simulink model "commhdlPRBSLoopback"  (R2025b)
settings: Solver=FixedStepDiscrete  StartTime=0.0  StopTime=5000  FixedStep=1  RelTol=1e-3
settings Model: Creator=tcollins  LastModifiedBy=tcollins

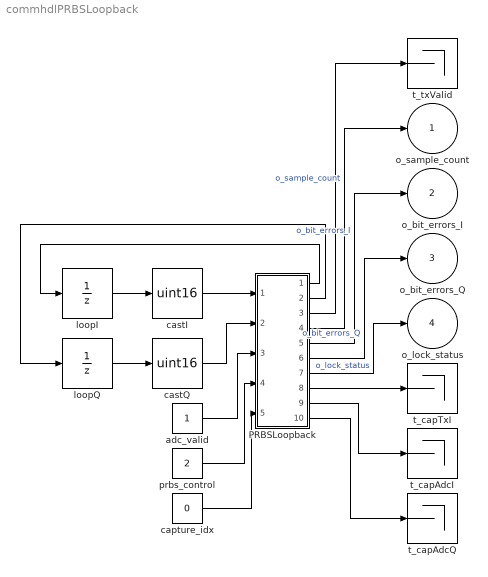
== system commhdlPRBSLoopback ==
  PRBSLoopback : Subsystem  TreatAsAtomicUnit=on
  adc_valid : Constant  OutDataTypeStr=boolean
  capture_idx : Constant  Value=0  OutDataTypeStr=uint32
  castI : DataTypeConversion  OutDataTypeStr=uint16
  castQ : DataTypeConversion  OutDataTypeStr=uint16
  loopI : UnitDelay
  loopQ : UnitDelay
  prbs_control : Constant  Value=2  OutDataTypeStr=uint32
  t_capAdcI : Terminator
  t_capAdcQ : Terminator
  t_capTxI : Terminator
  t_txValid : Terminator
  o_sample_count : Outport
  o_bit_errors_I : Outport  Port=2
  o_bit_errors_Q : Outport  Port=3
  o_lock_status : Outport  Port=4
  wires:
  PRBSLoopback/7(lock_status) -> o_lock_status/1  "o_lock_status"
  loopI/1 -> castI/1
  loopQ/1 -> castQ/1
  castI/1 -> PRBSLoopback/1(adc_dataInI)
  adc_valid/1 -> PRBSLoopback/3(adc_validIn)
  PRBSLoopback/10(capture_adcQ) -> t_capAdcQ/1
  castQ/1 -> PRBSLoopback/2(adc_dataInQ)
  prbs_control/1 -> PRBSLoopback/4(prbs_control)
  PRBSLoopback/3(tx_validOut) -> t_txValid/1
  capture_idx/1 -> PRBSLoopback/5(capture_idx)
  PRBSLoopback/8(capture_txI) -> t_capTxI/1
  PRBSLoopback/2(tx_dataOutQ) -> loopQ/1
  PRBSLoopback/1(tx_dataOutI) -> loopI/1
  PRBSLoopback/4(sample_count) -> o_sample_count/1  "o_sample_count"
  PRBSLoopback/5(bit_errors_I) -> o_bit_errors_I/1  "o_bit_errors_I"
  PRBSLoopback/9(capture_adcI) -> t_capAdcI/1
  PRBSLoopback/6(bit_errors_Q) -> o_bit_errors_Q/1  "o_bit_errors_Q"

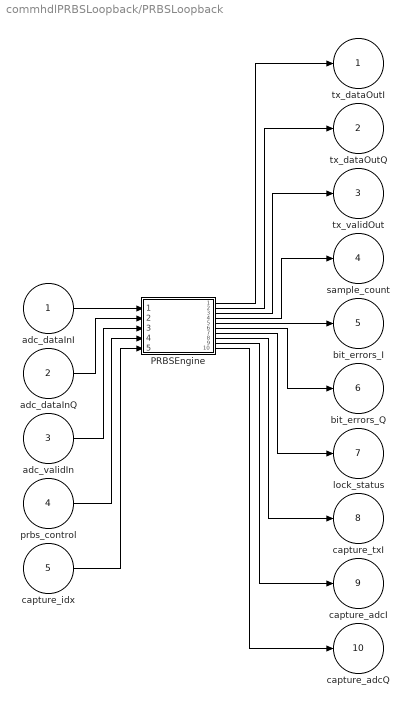
== system commhdlPRBSLoopback/PRBSLoopback ==
  adc_dataInI : Inport  OutDataTypeStr=uint16  PortDimensions=1
  adc_dataInQ : Inport  Port=2  OutDataTypeStr=uint16  PortDimensions=1
  adc_validIn : Inport  Port=3  OutDataTypeStr=boolean  PortDimensions=1
  prbs_control : Inport  Port=4  OutDataTypeStr=uint32  PortDimensions=1
  capture_idx : Inport  Port=5  OutDataTypeStr=uint32  PortDimensions=1
  PRBSEngine : MATLAB Function  TreatAsAtomicUnit=on
  tx_dataOutI : Outport
  tx_dataOutQ : Outport  Port=2
  tx_validOut : Outport  Port=3
  sample_count : Outport  Port=4
  bit_errors_I : Outport  Port=5
  bit_errors_Q : Outport  Port=6
  lock_status : Outport  Port=7
  capture_txI : Outport  Port=8
  capture_adcI : Outport  Port=9
  capture_adcQ : Outport  Port=10
  wires:
  PRBSEngine/10(capture_adcQ) -> capture_adcQ/1
  PRBSEngine/9(capture_adcI) -> capture_adcI/1
  PRBSEngine/6(bit_errors_Q) -> bit_errors_Q/1
  adc_dataInQ/1 -> PRBSEngine/2(adc_dataInQ)
  PRBSEngine/8(capture_txI) -> capture_txI/1
  prbs_control/1 -> PRBSEngine/4(prbs_control)
  capture_idx/1 -> PRBSEngine/5(capture_idx)
  adc_validIn/1 -> PRBSEngine/3(adc_validIn)
  PRBSEngine/3(tx_validOut) -> tx_validOut/1
  PRBSEngine/7(lock_status) -> lock_status/1
  PRBSEngine/2(tx_dataOutQ) -> tx_dataOutQ/1
  adc_dataInI/1 -> PRBSEngine/1(adc_dataInI)
  PRBSEngine/1(tx_dataOutI) -> tx_dataOutI/1
  PRBSEngine/4(sample_count) -> sample_count/1
  PRBSEngine/5(bit_errors_I) -> bit_errors_I/1

== matlab function commhdlPRBSLoopback/PRBSLoopback/PRBSEngine ==
  data: adc_dataInI input; tx_dataOutI output uint16 size=1; adc_dataInQ input; adc_validIn input; prbs_control input; capture_idx input; tx_dataOutQ output uint16 size=1; tx_validOut output boolean size=1; sample_count output uint32 size=1; bit_errors_I output uint32 size=1; bit_errors_Q output uint32 size=1; lock_status output uint8 size=1; capture_txI output uint16 size=1; capture_adcI output uint16 size=1; capture_adcQ output uint16 size=1
function [tx_dataOutI, tx_dataOutQ, tx_validOut, sample_count, bit_errors_I, bit_errors_Q, lock_status, capture_txI, capture_adcI, capture_adcQ] = prbs_loopback_step(adc_dataInI, adc_dataInQ, adc_validIn, prbs_control, capture_idx)
%#codegen
[tx_dataOutI, tx_dataOutQ, tx_validOut, sample_count, bit_errors_I, bit_errors_Q, lock_status, capture_txI, capture_adcI, capture_adcQ] = ...
    PRBSEngine(adc_dataInI, adc_dataInQ, adc_validIn, prbs_control, capture_idx);
end
